simulink model "PX11es"  (R2015b)
settings: Solver=VariableStepAuto  StartTime=0.0  StopTime=1  RelTol=1e-3
settings Model: Creator=xmax1946  LastModifiedBy=xmax1946

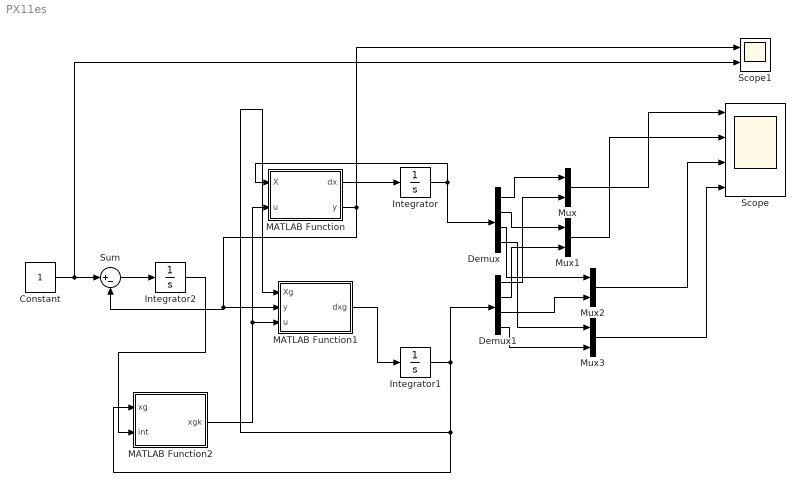
== system PX11es ==
  Constant : Constant
  Demux : Demux
  Demux1 : Demux
  Integrator : Integrator  InitialCondition=[0;0;0;0]
  Integrator1 : Integrator  InitialCondition=[.1;0.1;0.1;0.1]
  Integrator2 : Integrator  IgnoreLimit=on
  MATLAB Function : MATLAB Function  TreatAsAtomicUnit=on
  MATLAB Function1 : MATLAB Function  TreatAsAtomicUnit=on
  MATLAB Function2 : MATLAB Function  TreatAsAtomicUnit=on
  Mux{,1..3} (4 alike) : Mux  Inputs=2
  Scope : Scope  NumInputPorts=4
  Scope1 : Scope  NumInputPorts=2
  Sum : Sum  Inputs=|+-
  wires:
  MATLAB Function/1(dx) -> Integrator/1
  MATLAB Function1/1(dxg) -> Integrator1/1
  Integrator/1 -> MATLAB Function/1(X), Demux/1
  MATLAB Function/2(y) -> Sum/2, MATLAB Function1/2(y), Scope1/1
  Integrator1/1 -> MATLAB Function2/1(xg), MATLAB Function1/1(Xg), Demux1/1
  Demux/1 -> Mux/1
  Demux1/1 -> Mux/2
  Demux/2 -> Mux1/1
  Demux1/2 -> Mux1/2
  Mux/1 -> Scope/1
  Mux1/1 -> Scope/2
  Constant/1 -> Scope1/2, Sum/1
  Sum/1 -> Integrator2/1
  Integrator2/1 -> MATLAB Function2/2(int)
  MATLAB Function2/1(xgk) -> MATLAB Function/2(u), MATLAB Function1/3(u)
  Demux/3 -> Mux2/1
  Demux/4 -> Mux3/1
  Demux1/3 -> Mux2/2
  Demux1/4 -> Mux3/2
  Mux2/1 -> Scope/3
  Mux3/1 -> Scope/4

== matlab function PX11es/MATLAB Function1 ==
  data: Xg input; y input; u input; dxg output
function dxg =fcn(Xg,y,u)
A=[400,-899,1409,-399;200,-450,704,-198;0,0,0,1;0,1,0,0];
B=[1;0;0;1];
C=[1,-2,3,-1];

L=[3.6916;.5209;.1344;3.0509]*1e+05;
dxg=A*Xg+B*u+L*(y-C*Xg);

== matlab function PX11es/MATLAB Function ==
  data: dx output; X input; y output; u input
function [dx,y]=fcn(X,u)
A=[400,-899,1409,-399;200,-450,704,-198;0,0,0,1;0,1,0,0];
B=[1;0;0;1];
C=[1,-2,3,-1];
dx=A*X+B*u;
y=C*X;

== matlab function PX11es/MATLAB Function2 ==
  data: xg input; xgk output; int input
function xgk = fcn(xg,int)
ki=1.517279174657143e+06;
K=[2.0964,-4.327,6.6545,-2.0945]*1e+05;
xgk=int*ki-K*xg;
